simulink model "inverter_simulation"  (R2024b)
settings: Solver=VariableStepAuto  StartTime=0.0  StopTime=2  RelTol=1e-3
values from neighbouring files (symbols this model uses):
  Cdc = 2200e-6    (= 0.0022)    [parameters.m]
  KI_curr_d = KP_curr_d * Wp1_in    [pi_tuning.m]
  KI_curr_q = KI_curr_d    [pi_tuning.m]
  KI_q = C_q_ctrl.Ki    [pi_tuning.m]
  KI_volt = C_volt.Ki    [pi_tuning.m]
  KP_curr_d = Wbi / (DCGain_id * Wp1_in)    [pi_tuning.m]
  KP_curr_q = KP_curr_d    [pi_tuning.m]
  KP_q = C_q_ctrl.Kp    [pi_tuning.m]
  KP_volt = C_volt.Kp    [pi_tuning.m]
  Lc = 2.54e-3    (= 0.00254)    [parameters.m]
  P = 0.041    [parameters.m]
  rac = 1e-3    (= 0.001)    [parameters.m]
  rdc = Vdc^2 / P    (= 21951.2195122)    [parameters.m]
  Vdc = 30    [parameters.m]
  Vs = 20/sqrt(2)    [parameters.m]
  Zl = w * Lc    (= 0.957557440814)    [parameters.m]
libraries: slpidlib x4, spsMosfetLib x4, spsSeriesRLCBranchLib x3, spsVoltageMeasurementLib x3, spsCurrentMeasurementLib x2, spsACVoltageSourceLib x1, spsParallelRLCBranchLib x1, spsGroundLib x1, spsPWMGenerator2LevelLib x1, eePowerMeasurement x1, spspowerguiLib x1
settings Model: Creator=Asus  LastModifiedBy=Asus
settings RTWCC: GenCodeOnly=on

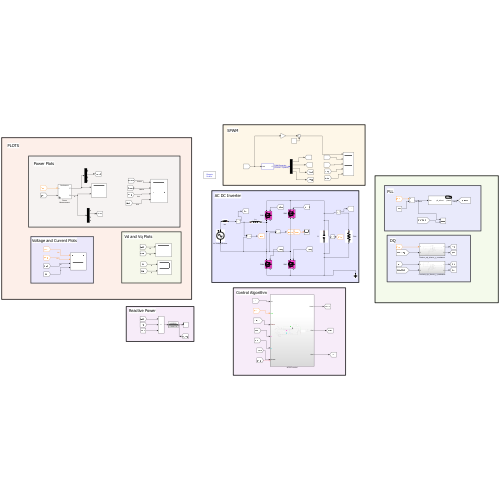
[thumbnail: Simulink's stored preview of the top-level diagram]
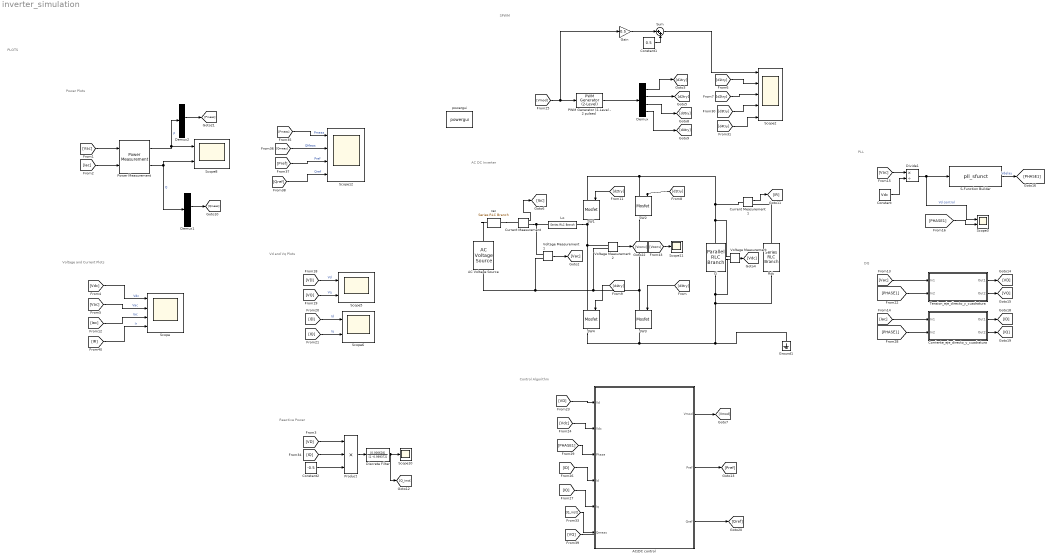
== system inverter_simulation ==
  note: PLL
  note: SPWM
  note: PLOTS
  note: Control Algorithm
  note: AC DC Inverter
  note: Power Plots
  note: Voltage and Current Plots
  note: Vd and Vq Plots
  note: DQ
  note: Reactive Power
  AC Voltage Source : spsACVoltageSourceLib/AC Voltage Source  Amplitude=Vs*sqrt(2)  Phase=0  Frequency=60  SampleTime=0  Measurements=None  BusType=swing  Pref=10e3  Qref=0  Qmin=-inf  Qmax=+inf
  AC/DC control : Subsystem
  Ci : spsParallelRLCBranchLib/Parallel RLC Branch  LConnTagsString=a  RConnTagsString=__new0  BranchType=C  Resistance=1  Inductance=1e-3  SetiL0=off  InitialCurrent=0  Capacitance=Cdc  Setx0=on  InitialVoltage=20  Measurements=None
  Constant : Constant  Value=Vdc
  Constant1 : Constant  Value=0.5
  Constant2 : Constant  Value=-0.5
  Corriente_eje_directo_y_cuadratura : Subsystem
  Current Measurement : spsCurrentMeasurementLib/Current Measurement  PhasorSimulation=off  OutputType=Complex  PSBequivalent=0
  Current Measurement1 : spsCurrentMeasurementLib/Current Measurement  PhasorSimulation=off  OutputType=Complex  PSBequivalent=0
  Demux : Demux
  Demux1 : Demux
  Demux2 : Demux
  Discrete Filter : DiscreteFilter  Numerator=[0.000628]  Denominator=[1 -0.999372]
  Divide1 : Product  Inputs=*/
  Gain : Gain  Gain=0.5
  Ground1 : spsGroundLib/Ground  LConnTagsString=a
  Lo : spsSeriesRLCBranchLib/Series RLC Branch  LConnTagsString=__new0  RConnTagsString=__new0  BranchType=L  Resistance=rac  Inductance=Lc  SetiL0=off  InitialCurrent=Io0  Capacitance=1e-6  Setx0=off  InitialVoltage=0  Measurements=None
  PWM Generator (2-Level - 2 pulses) : spsPWMGenerator2LevelLib/PWM Generator (2-Level)  ModulatorType=Single-phase full-bridge - Bipolar modulation (4 pulses)  ModulatorMode=Unsynchronized  Fc=20000  Pc=0  nF=27  MinMax="[ -1  1 ]"  SamplingTechnique=Natural  ModulatingSignals=off  m=0.6  Freq=60  Phase=30  Ts=5e-6  ShowCarrierOutport=off
  Power Measurement : eePowerMeasurement/Power Measurement  LabelModeActiveChoice=Continuous  F=60  K=[0 1 2 3]  Ts=0
  Product : Product  Inputs=3
  Rdc : spsSeriesRLCBranchLib/Series RLC Branch  LConnTagsString=__new0  RConnTagsString=__new0  BranchType=R  Resistance=rdc  Inductance=1e-3  SetiL0=off  InitialCurrent=0  Capacitance=1e-6  Setx0=off  InitialVoltage=0  Measurements=None
  S-Function Builder : S-Function  FunctionName=pll_sfunct  SFunctionModules=pll_sfunct_wrapper.c  SFunctionDeploymentMode=off  EnableBusSupport=off  mask(S-Function Builder){}
      mask help: Simulink:masks:SFunctionBuilder_MD
      mask init:
      | val = [[.9  0.75 0.75 1 1 .9 .9 1]',[1 1 0.75 0.75 .9 .9 1 .9]'];try , sys = get_param(gcb,'SfunBuilderFcnName');if isempty(sys), sys = get_param(gcb,'FunctionName'); end,catch, sys = get_param(gcb,'FunctionName'); end
      settings: CopyFcn=set_param(gcbh,'LinkStatus','none')  OpenFcn=sfunctionwizard(gcbh)
      mask Display:
      | plot(val(:,1),val(:,2))
      | disp(sys)
      | port_label('input',1,sprintf('%s', 'Vac'),'interpreter','tex')
      | port_label('output',1,sprintf('%s', 'phase'),'interpreter','tex')
  SW{1..4} (4 alike) : spsMosfetLib/Mosfet  Ron=1e-3  Lon=0  Rd=0.00001  Vfd=0  IC=0  Rs=1e5  Cs=inf  Measurements=on
  Scope : Scope  NumInputPorts=4
  Scope10 : Scope
  Scope11 : Scope
  Scope12 : Scope  NumInputPorts=4
  Scope2 : Scope  NumInputPorts=5
  Scope{3,5..6,8} (4 alike) : Scope  NumInputPorts=2
  Sum : Sum  Inputs=|++
  Tension_eje_directo_y_cuadratura : Subsystem
  Voltage Measurement : spsVoltageMeasurementLib/Voltage Measurement  PhasorSimulation=off  OutputType=Complex  PSBequivalent=0
  Voltage Measurement1 : spsVoltageMeasurementLib/Voltage Measurement  PhasorSimulation=off  OutputType=Complex  PSBequivalent=0
  Voltage Measurement2 : spsVoltageMeasurementLib/Voltage Measurement  PhasorSimulation=off  OutputType=Complex  PSBequivalent=0
  powergui : spspowerguiLib/powergui  Priority=1  SimulationMode=Discrete  SampleTime=5e-6  frequency=60  Iterations=50  frequencyindice=60  Pbase=100e6  ErrMax=1e-4  UnitsV=kV  UnitsW=MW  buscounter=0  FunctionMessages=off  echomessages=off  EnableUseOfTLC=off  CurrentSourceSwitches=off  DisableSnubberDevices=off  DisableRonSwitches=off  DisableVfSwitches=off  DisplayEquations=off  AutomaticDiscreteSolvers=off  SolverType=Tustin/Backward Euler (TBE)  Interpol=off  ExternalGateDelay=off  methode=off  Ts=100  x0status=blocks  SPID=on  SwTol=0  HookPort=off  NonlinearTolerance=1e-4  nMaxIteration=100  ContinueOnMaxIteration=off  RestoreLinks=warning  ResistiveCurrentMeasurement=off  Frange=[0:2:500]  Ylog=off  Xlog=on  ShowGrid=off  save=off  variable=ZData  structure=0  ZoomFFT=off  StartTime=0.0  cycles=1  DisplayStyle=1  fundamental=60  FreqAxis=off  MaxFrequency=1000  frequencyindicesteady=1  RmsSteady=1  display=off
  rac : spsSeriesRLCBranchLib/Series RLC Branch  LConnTagsString=__new0  RConnTagsString=__new0  BranchType=R  Resistance=rac  Inductance=Lc  SetiL0=off  InitialCurrent=Io0  Capacitance=1e-6  Setx0=off  InitialVoltage=0  Measurements=None
  wires:
  Voltage Measurement/1 -> [Vdc]
  PWM Generator (2-Level - 2 pulses)/1 -> Demux/1
  Demux/1 -> [d1try]
  Demux/2 -> [d2try]
  [d1try] -> Scope2/2
  [d2try] -> Scope2/3
  Current Measurement/1 -> [Iac]
  Tension_eje_directo_y_cuadratura/1(Out1) -> [VD]
  Corriente_eje_directo_y_cuadratura/1(Out1) -> [ID]
  Tension_eje_directo_y_cuadratura/2(Out2) -> [VQ]
  [Iac] -> Corriente_eje_directo_y_cuadratura/1(In1)
  [Vac] -> Tension_eje_directo_y_cuadratura/1(In1)
  [PHASE1] -> Corriente_eje_directo_y_cuadratura/2(In2)
  Corriente_eje_directo_y_cuadratura/2(Out2) -> [IQ]
  [PHASE1] -> Tension_eje_directo_y_cuadratura/2(In2)
  [PHASE1] -> Scope3/2
  [VD] -> Scope5/1  "Vd"
  [VQ] -> Scope5/2  "Vq"
  [ID] -> Scope6/1  "Id"
  [IQ] -> Scope6/2  "Iq"
  [VD] -> AC/DC control/1(Vd)
  [Vdc] -> AC/DC control/2(Vdc)
  AC/DC control/1(Vmod) -> [Vmod]
  [PHASE1] -> AC/DC control/3(Phase)
  [Vac] -> Divide1/1
  Divide1/1 -> Scope3/1, S-Function Builder/1  "Vd control"
  Constant/1 -> Divide1/2
  Demux/3 -> [d3try]
  Demux/4 -> [d4try]
  [d3try] -> Scope2/4
  [d4try] -> Scope2/5
  Voltage Measurement1/1 -> [Vac]
  [ID] -> AC/DC control/4(Id)
  [IQ] -> AC/DC control/5(Iq)
  Current Measurement1/1 -> [IR]
  Voltage Measurement2/1 -> [Vconv]
  [Vconv] -> Scope11/1
  [d1try] -> SW2/1
  [d2try] -> SW1/1
  [d4try] -> SW4/1
  Gain/1 -> Sum/1
  Constant1/1 -> Sum/2
  Sum/1 -> Scope2/1
  [d3try] -> SW3/1
  S-Function Builder/1 -> [PHASE1]  "Vdelay"
  Constant2/1 -> Product/3
  [IQ] -> Product/2
  Discrete Filter/1 -> [Q_inst], Scope10/1
  [VD] -> Product/1
  Product/1 -> Discrete Filter/1
  [Q_inst] -> AC/DC control/6(Qmeas)
  AC/DC control/2(Pref) -> [Pref]
  AC/DC control/3(Qref) -> [Qref]
  [VQ] -> ?
  [Vmod] -> Gain/1, PWM Generator (2-Level - 2 pulses)/1
  [IR] -> Scope/4  "Ir"
  [Pref] -> Scope12/3  "Pref"
  [Iac] -> Scope/3  "Iac"
  [Qref] -> Scope12/4  "Qref"
  [Qmeas] -> Scope12/2  "QMeas"
  [Vac] -> Scope/2  "Vac"
  [Vac] -> Power Measurement/1
  Power Measurement/1 -> Demux2/1, Scope8/1  "P"
  [Vdc] -> Scope/1  "Vdc"
  Power Measurement/2 -> Demux1/1, Scope8/2  "Q"
  [Iac] -> Power Measurement/2
  Demux1/2 -> [Qmeas]
  [Pmeas] -> Scope12/1  "Pmeas"
  Demux2/2 -> [Pmeas]
  connections:
  Current Measurement/RConn1 -- Voltage Measurement1/LConn1 -- Lo/LConn1
  SW1/LConn1 -- Ci/LConn1 -- Voltage Measurement/LConn1 -- Current Measurement1/LConn1 -- SW2/LConn1
  Ci/RConn1 -- Voltage Measurement/LConn2 -- SW3/RConn1 -- SW4/RConn1 -- Ground1/LConn1 -- Rdc/RConn1
  SW2/RConn1 -- Voltage Measurement2/LConn2 -- AC Voltage Source/LConn1 -- Voltage Measurement1/LConn2 -- SW3/LConn1
  Lo/RConn1 -- Voltage Measurement2/LConn1 -- SW4/LConn1 -- SW1/RConn1
  rac/RConn1 -- AC Voltage Source/RConn1
  rac/LConn1 -- Current Measurement/LConn1
  Rdc/LConn1 -- Current Measurement1/RConn1

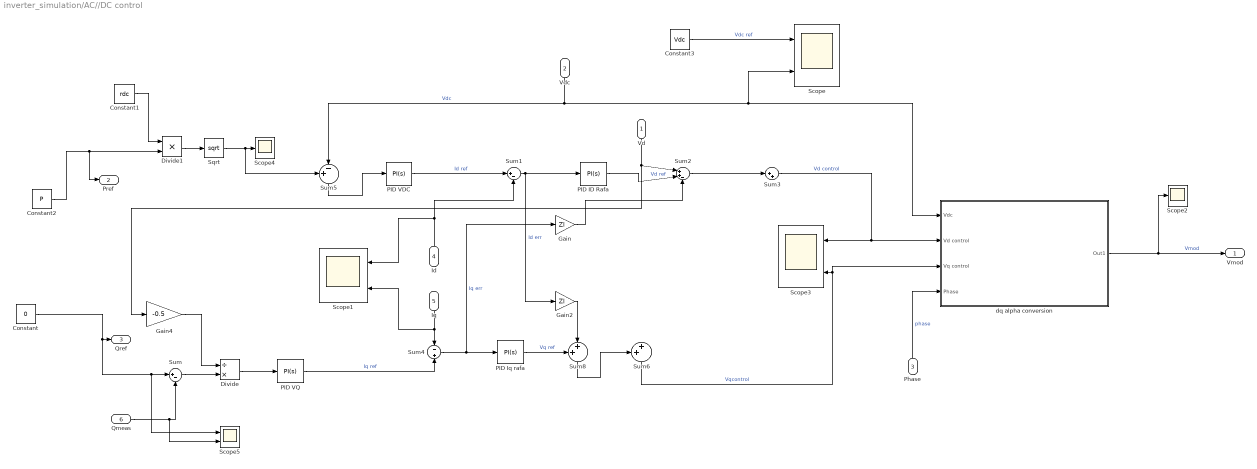
== system inverter_simulation/AC//DC control ==
  Vd : Inport
  Vdc : Inport  Port=2
  Phase : Inport  Port=3
  Id : Inport  Port=4
  Iq : Inport  Port=5
  Qmeas : Inport  Port=6
  Constant : Constant  Value=0
  Constant1 : Constant  Value=rdc
  Constant2 : Constant  Value=P
  Constant3 : Constant  Value=Vdc
  Divide : Product  Inputs=/*
  Divide1 : Product  Inputs=**
  Gain : Gain  Gain=Zl
  Gain2 : Gain  Gain=Zl
  Gain4 : Gain  Gain=-0.5
  PID ID Rafa : slpidlib/PID Controller  Controller=PI  Form=Parallel  TimeDomain=Continuous-time  UseExternalTs=off  SampleTime=-1  IntegratorMethod=Forward Euler  FilterMethod=Forward Euler  ControllerParametersSource=internal  P=KP_curr_d  I=KI_curr_d  UseKiTs=off  D=0  UseExternalDerivativeSource=off  N=100  UseFilter=on  TunerSelectOption=Transfer Function Based (PID Tuner App)  InitialConditionSource=internal  InitialConditionForIntegrator=0  InitialConditionForFilter=0  DifferentiatorICPrevScaledInput=0  ExternalReset=none  TrackingMode=off  Kt=1  LimitOutput=off  SatLimitsSource=internal  UpperSaturationLimit=200  LowerSaturationLimit=-inf  LinearizeAsGain=on  AntiWindupMode=none  Kb=1  LimitIntegrator=off  UpperIntegratorSaturationLimit=inf  LowerIntegratorSaturationLimit=-inf  POutMin=[]  POutMax=[]  IOutMin=[]  IOutMax=[]  DOutMin=[]  DOutMax=[]  NOutMin=[]  NOutMax=[]  SumOutMin=[]  SumOutMax=[]  SaturationOutMin=[]  SaturationOutMax=[]  PParamMin=[]  PParamMax=[]  IParamMin=[]  IParamMax=[]  DParamMin=[]  DParamMax=[]  NParamMin=[]  NParamMax=[]  KbParamMin=[]  KbParamMax=[]  KtParamMin=[]  KtParamMax=[]  KbOutMin=[]  KbOutMax=[]  KtOutMin=[]  KtOutMax=[]  IntegratorOutMin=[]  IntegratorOutMax=[]  FilterOutMin=[]  FilterOutMax=[]  SumI1OutMin=[]  SumI1OutMax=[]  SumI2OutMin=[]  SumI2OutMax=[]  SumI3OutMin=[]  SumI3OutMax=[]  SumI4OutMin=[]  SumI4OutMax=[]  SumDOutMin=[]  SumDOutMax=[]  DifferentiatorOutMin=[]  DifferentiatorOutMax=[]  FilterDiffOutCoefMin=[]  FilterDiffOutCoefMax=[]  ReciprocalOutMin=[]  ReciprocalOutMax=[]  SumDenOutMin=[]  SumDenOutMax=[]  SumNumOutMin=[]  SumNumOutMax=[]  DivideOutMin=[]  DivideOutMax=[]  UdiffTsProdOutMin=[]  UdiffTsProdOutMax=[]  NTsProdOutMin=[]  NTsProdOutMax=[]  UintegralTsProdOutMin=[]  UintegralTsProdOutMax=[]  UngainTsProdOutMin=[]  UngainTsProdOutMax=[]  ClampingZeroOutDataTypeStr=Inherit: Inherit via back propagation  ClampingZeroOutMin=[]  ClampingZeroOutMax=[]  FilterDenConstantOutDataTypeStr=Inherit: Inherit via back propagation  FilterDenConstantOutMin=[]  FilterDenConstantOutMax=[]  PCopyOutDataTypeStr=Inherit: Inherit via back propagation  PCopyOutMin=[]  PCopyOutMax=[]  NCopyOutDataTypeStr=Inherit: Inherit via back propagation  NCopyOutMin=[]  NCopyOutMax=[]  IntegratorContinuousStateAttributes=''  IntegratorStateMustResolveToSignalObject=off  IntegratorRTWStateStorageClass=Auto  FilterContinuousStateAttributes=''  FilterStateMustResolveToSignalObject=off  FilterRTWStateStorageClass=Auto  ParallelPVariant=InternalParameters  IdealPVariant=Disabled  IVariant=InternalParameters  DVariant=Disabled  IntegratorVariant=Continuous  SatVariant=Disabled  AWVariant=Passthrough  PCopyVariant=Disabled  TRVariant=Disabled  FdbkBlocksVariant=Forward  IdealPFdbkVariant=Disabled  SatFdbkVariant=Disabled  DerivativeFilterVariant=Disabled  NVariant=Disabled  NCopyVariant=Disabled_SignalSpec  FilterICVariant=Disabled  IntegratorICVariant=InternalICs  ExternalResetVariant=Disabled  TRSumVariant=Passthrough  SumFdbkVariant=Disabled  SumVariant=Sum_PI  TsampFilterVariant=InternalTs  TsampNgainVariant=Passthrough  TsampIntegralVariant=Disabled_SignalSpec  ExternalSaturationOutDataTypeStr=Inherit: Same as second input  DerivativeSourceVariant=Disabled  PreIntVariant=InternalPreInt
  PID Iq rafa : slpidlib/PID Controller  Controller=PI  Form=Parallel  TimeDomain=Continuous-time  UseExternalTs=off  SampleTime=-1  IntegratorMethod=Forward Euler  FilterMethod=Forward Euler  ControllerParametersSource=internal  P=KP_curr_q  I=KI_curr_q  UseKiTs=off  D=0  UseExternalDerivativeSource=off  N=100  UseFilter=on  TunerSelectOption=Transfer Function Based (PID Tuner App)  InitialConditionSource=internal  InitialConditionForIntegrator=0  InitialConditionForFilter=0  DifferentiatorICPrevScaledInput=0  ExternalReset=none  TrackingMode=off  Kt=1  LimitOutput=off  SatLimitsSource=internal  UpperSaturationLimit=15  LowerSaturationLimit=-15  LinearizeAsGain=on  AntiWindupMode=none  Kb=1  LimitIntegrator=off  UpperIntegratorSaturationLimit=inf  LowerIntegratorSaturationLimit=-inf  POutMin=[]  POutMax=[]  IOutMin=[]  IOutMax=[]  DOutMin=[]  DOutMax=[]  NOutMin=[]  NOutMax=[]  SumOutMin=[]  SumOutMax=[]  SaturationOutMin=[]  SaturationOutMax=[]  PParamMin=[]  PParamMax=[]  IParamMin=[]  IParamMax=[]  DParamMin=[]  DParamMax=[]  NParamMin=[]  NParamMax=[]  KbParamMin=[]  KbParamMax=[]  KtParamMin=[]  KtParamMax=[]  KbOutMin=[]  KbOutMax=[]  KtOutMin=[]  KtOutMax=[]  IntegratorOutMin=[]  IntegratorOutMax=[]  FilterOutMin=[]  FilterOutMax=[]  SumI1OutMin=[]  SumI1OutMax=[]  SumI2OutMin=[]  SumI2OutMax=[]  SumI3OutMin=[]  SumI3OutMax=[]  SumI4OutMin=[]  SumI4OutMax=[]  SumDOutMin=[]  SumDOutMax=[]  DifferentiatorOutMin=[]  DifferentiatorOutMax=[]  FilterDiffOutCoefMin=[]  FilterDiffOutCoefMax=[]  ReciprocalOutMin=[]  ReciprocalOutMax=[]  SumDenOutMin=[]  SumDenOutMax=[]  SumNumOutMin=[]  SumNumOutMax=[]  DivideOutMin=[]  DivideOutMax=[]  UdiffTsProdOutMin=[]  UdiffTsProdOutMax=[]  NTsProdOutMin=[]  NTsProdOutMax=[]  UintegralTsProdOutMin=[]  UintegralTsProdOutMax=[]  UngainTsProdOutMin=[]  UngainTsProdOutMax=[]  ClampingZeroOutDataTypeStr=Inherit: Inherit via back propagation  ClampingZeroOutMin=[]  ClampingZeroOutMax=[]  FilterDenConstantOutDataTypeStr=Inherit: Inherit via back propagation  FilterDenConstantOutMin=[]  FilterDenConstantOutMax=[]  PCopyOutDataTypeStr=Inherit: Inherit via back propagation  PCopyOutMin=[]  PCopyOutMax=[]  NCopyOutDataTypeStr=Inherit: Inherit via back propagation  NCopyOutMin=[]  NCopyOutMax=[]  IntegratorContinuousStateAttributes=''  IntegratorStateMustResolveToSignalObject=off  IntegratorRTWStateStorageClass=Auto  FilterContinuousStateAttributes=''  FilterStateMustResolveToSignalObject=off  FilterRTWStateStorageClass=Auto  ParallelPVariant=InternalParameters  IdealPVariant=Disabled  IVariant=InternalParameters  DVariant=Disabled  IntegratorVariant=Continuous  SatVariant=Disabled  AWVariant=Passthrough  PCopyVariant=Disabled  TRVariant=Disabled  FdbkBlocksVariant=Forward  IdealPFdbkVariant=Disabled  SatFdbkVariant=Disabled  DerivativeFilterVariant=Disabled  NVariant=Disabled  NCopyVariant=Disabled_SignalSpec  FilterICVariant=Disabled  IntegratorICVariant=InternalICs  ExternalResetVariant=Disabled  TRSumVariant=Passthrough  SumFdbkVariant=Disabled  SumVariant=Sum_PI  TsampFilterVariant=InternalTs  TsampNgainVariant=Passthrough  TsampIntegralVariant=Disabled_SignalSpec  ExternalSaturationOutDataTypeStr=Inherit: Same as second input  DerivativeSourceVariant=Disabled  PreIntVariant=InternalPreInt
  PID VDC : slpidlib/PID Controller  Controller=PI  Form=Parallel  TimeDomain=Continuous-time  UseExternalTs=off  SampleTime=-1  IntegratorMethod=Forward Euler  FilterMethod=Forward Euler  ControllerParametersSource=internal  P=-KP_volt  I=-KI_volt  UseKiTs=off  D=0  UseExternalDerivativeSource=off  N=100  UseFilter=on  TunerSelectOption=Frequency Response Based  InitialConditionSource=internal  InitialConditionForIntegrator=0  InitialConditionForFilter=0  DifferentiatorICPrevScaledInput=0  ExternalReset=none  TrackingMode=off  Kt=1  LimitOutput=off  SatLimitsSource=internal  UpperSaturationLimit=16  LowerSaturationLimit=-16  LinearizeAsGain=on  AntiWindupMode=none  Kb=1  LimitIntegrator=off  UpperIntegratorSaturationLimit=inf  LowerIntegratorSaturationLimit=-inf  POutMin=[]  POutMax=[]  IOutMin=[]  IOutMax=[]  DOutMin=[]  DOutMax=[]  NOutMin=[]  NOutMax=[]  SumOutMin=[]  SumOutMax=[]  SaturationOutMin=[]  SaturationOutMax=[]  PParamMin=[]  PParamMax=[]  IParamMin=[]  IParamMax=[]  DParamMin=[]  DParamMax=[]  NParamMin=[]  NParamMax=[]  KbParamMin=[]  KbParamMax=[]  KtParamMin=[]  KtParamMax=[]  KbOutMin=[]  KbOutMax=[]  KtOutMin=[]  KtOutMax=[]  IntegratorOutMin=[]  IntegratorOutMax=[]  FilterOutMin=[]  FilterOutMax=[]  SumI1OutMin=[]  SumI1OutMax=[]  SumI2OutMin=[]  SumI2OutMax=[]  SumI3OutMin=[]  SumI3OutMax=[]  SumI4OutMin=[]  SumI4OutMax=[]  SumDOutMin=[]  SumDOutMax=[]  DifferentiatorOutMin=[]  DifferentiatorOutMax=[]  FilterDiffOutCoefMin=[]  FilterDiffOutCoefMax=[]  ReciprocalOutMin=[]  ReciprocalOutMax=[]  SumDenOutMin=[]  SumDenOutMax=[]  SumNumOutMin=[]  SumNumOutMax=[]  DivideOutMin=[]  DivideOutMax=[]  UdiffTsProdOutMin=[]  UdiffTsProdOutMax=[]  NTsProdOutMin=[]  NTsProdOutMax=[]  UintegralTsProdOutMin=[]  UintegralTsProdOutMax=[]  UngainTsProdOutMin=[]  UngainTsProdOutMax=[]  ClampingZeroOutDataTypeStr=Inherit: Inherit via back propagation  ClampingZeroOutMin=[]  ClampingZeroOutMax=[]  FilterDenConstantOutDataTypeStr=Inherit: Inherit via back propagation  FilterDenConstantOutMin=[]  FilterDenConstantOutMax=[]  PCopyOutDataTypeStr=Inherit: Inherit via back propagation  PCopyOutMin=[]  PCopyOutMax=[]  NCopyOutDataTypeStr=Inherit: Inherit via back propagation  NCopyOutMin=[]  NCopyOutMax=[]  IntegratorContinuousStateAttributes=''  IntegratorStateMustResolveToSignalObject=off  IntegratorRTWStateStorageClass=Auto  FilterContinuousStateAttributes=''  FilterStateMustResolveToSignalObject=off  FilterRTWStateStorageClass=Auto  ParallelPVariant=InternalParameters  IdealPVariant=Disabled  IVariant=InternalParameters  DVariant=Disabled  IntegratorVariant=Continuous  SatVariant=Disabled  AWVariant=Passthrough  PCopyVariant=Disabled  TRVariant=Disabled  FdbkBlocksVariant=Forward  IdealPFdbkVariant=Disabled  SatFdbkVariant=Disabled  DerivativeFilterVariant=Disabled  NVariant=Disabled  NCopyVariant=Disabled_SignalSpec  FilterICVariant=Disabled  IntegratorICVariant=InternalICs  ExternalResetVariant=Disabled  TRSumVariant=Passthrough  SumFdbkVariant=Disabled  SumVariant=Sum_PI  TsampFilterVariant=InternalTs  TsampNgainVariant=Passthrough  TsampIntegralVariant=Disabled_SignalSpec  ExternalSaturationOutDataTypeStr=Inherit: Same as second input  DerivativeSourceVariant=Disabled  PreIntVariant=InternalPreInt
  PID VQ : slpidlib/PID Controller  Controller=PI  Form=Parallel  TimeDomain=Continuous-time  UseExternalTs=off  SampleTime=-1  IntegratorMethod=Forward Euler  FilterMethod=Forward Euler  ControllerParametersSource=internal  P=KP_q+0.08  I=KI_q  UseKiTs=off  D=0  UseExternalDerivativeSource=off  N=100  UseFilter=on  TunerSelectOption=Frequency Response Based  InitialConditionSource=internal  InitialConditionForIntegrator=0  InitialConditionForFilter=0  DifferentiatorICPrevScaledInput=0  ExternalReset=none  TrackingMode=off  Kt=1  LimitOutput=off  SatLimitsSource=internal  UpperSaturationLimit=16  LowerSaturationLimit=-16  LinearizeAsGain=on  AntiWindupMode=none  Kb=1  LimitIntegrator=off  UpperIntegratorSaturationLimit=inf  LowerIntegratorSaturationLimit=-inf  POutMin=[]  POutMax=[]  IOutMin=[]  IOutMax=[]  DOutMin=[]  DOutMax=[]  NOutMin=[]  NOutMax=[]  SumOutMin=[]  SumOutMax=[]  SaturationOutMin=[]  SaturationOutMax=[]  PParamMin=[]  PParamMax=[]  IParamMin=[]  IParamMax=[]  DParamMin=[]  DParamMax=[]  NParamMin=[]  NParamMax=[]  KbParamMin=[]  KbParamMax=[]  KtParamMin=[]  KtParamMax=[]  KbOutMin=[]  KbOutMax=[]  KtOutMin=[]  KtOutMax=[]  IntegratorOutMin=[]  IntegratorOutMax=[]  FilterOutMin=[]  FilterOutMax=[]  SumI1OutMin=[]  SumI1OutMax=[]  SumI2OutMin=[]  SumI2OutMax=[]  SumI3OutMin=[]  SumI3OutMax=[]  SumI4OutMin=[]  SumI4OutMax=[]  SumDOutMin=[]  SumDOutMax=[]  DifferentiatorOutMin=[]  DifferentiatorOutMax=[]  FilterDiffOutCoefMin=[]  FilterDiffOutCoefMax=[]  ReciprocalOutMin=[]  ReciprocalOutMax=[]  SumDenOutMin=[]  SumDenOutMax=[]  SumNumOutMin=[]  SumNumOutMax=[]  DivideOutMin=[]  DivideOutMax=[]  UdiffTsProdOutMin=[]  UdiffTsProdOutMax=[]  NTsProdOutMin=[]  NTsProdOutMax=[]  UintegralTsProdOutMin=[]  UintegralTsProdOutMax=[]  UngainTsProdOutMin=[]  UngainTsProdOutMax=[]  ClampingZeroOutDataTypeStr=Inherit: Inherit via back propagation  ClampingZeroOutMin=[]  ClampingZeroOutMax=[]  FilterDenConstantOutDataTypeStr=Inherit: Inherit via back propagation  FilterDenConstantOutMin=[]  FilterDenConstantOutMax=[]  PCopyOutDataTypeStr=Inherit: Inherit via back propagation  PCopyOutMin=[]  PCopyOutMax=[]  NCopyOutDataTypeStr=Inherit: Inherit via back propagation  NCopyOutMin=[]  NCopyOutMax=[]  IntegratorContinuousStateAttributes=''  IntegratorStateMustResolveToSignalObject=off  IntegratorRTWStateStorageClass=Auto  FilterContinuousStateAttributes=''  FilterStateMustResolveToSignalObject=off  FilterRTWStateStorageClass=Auto  ParallelPVariant=InternalParameters  IdealPVariant=Disabled  IVariant=InternalParameters  DVariant=Disabled  IntegratorVariant=Continuous  SatVariant=Disabled  AWVariant=Passthrough  PCopyVariant=Disabled  TRVariant=Disabled  FdbkBlocksVariant=Forward  IdealPFdbkVariant=Disabled  SatFdbkVariant=Disabled  DerivativeFilterVariant=Disabled  NVariant=Disabled  NCopyVariant=Disabled_SignalSpec  FilterICVariant=Disabled  IntegratorICVariant=InternalICs  ExternalResetVariant=Disabled  TRSumVariant=Passthrough  SumFdbkVariant=Disabled  SumVariant=Sum_PI  TsampFilterVariant=InternalTs  TsampNgainVariant=Passthrough  TsampIntegralVariant=Disabled_SignalSpec  ExternalSaturationOutDataTypeStr=Inherit: Same as second input  DerivativeSourceVariant=Disabled  PreIntVariant=InternalPreInt
  Scope{,1,3,5} (4 alike) : Scope  NumInputPorts=2
  Scope2 : Scope
  Scope4 : Scope
  Sqrt : Sqrt
  Sum : Sum  Inputs=|+-
  Sum1 : Sum  Inputs=|+-
  Sum2 : Sum  Inputs=|++-
  Sum3 : Sum  Inputs=|++
  Sum4 : Sum  Inputs=-+
  Sum5 : Sum  Inputs=+-|
  Sum6 : Sum  Inputs=++|
  Sum8 : Sum  Inputs=++|
  dq alpha conversion : Subsystem
  Vmod : Outport
  Pref : Outport  Port=2
  Qref : Outport  Port=3
  wires:
  Sum4/1 -> PID Iq rafa/1, Gain/1  "Iq err"
  Sum8/1 -> Sum6/1
  Sum1/1 -> PID ID Rafa/1, Gain2/1  "Id err"
  Sum2/1 -> Sum3/1
  PID Iq rafa/1 -> Sum8/1  "Vq ref"
  Phase/1 -> dq alpha conversion/4(Phase)  "phase"
  PID ID Rafa/1 -> Sum2/2  "Vd ref"
  Vdc/1 -> Scope/2, dq alpha conversion/1(Vdc), Sum5/2  "Vdc"
  dq alpha conversion/1(Out1) -> Scope2/1, Vmod/1  "Vmod"
  Sum5/1 -> PID VDC/1
  Gain/1 -> Sum2/3
  Gain2/1 -> Sum8/2
  Id/1 -> Scope1/1, Sum1/2
  Iq/1 -> Scope1/2, Sum4/1
  Sum3/1 -> Scope3/1, dq alpha conversion/2(Vd control)  "Vd control"
  Sum6/1 -> dq alpha conversion/3(Vq control), Scope3/2  "Vqcontrol"
  Constant3/1 -> Scope/1  "Vdc ref"
  Vd/1 -> Gain4/1, Sum2/1
  Divide/1 -> PID VQ/1
  Qmeas/1 -> Scope5/2, Sum/2
  Sum/1 -> Divide/2
  Gain4/1 -> Divide/1
  Constant/1 -> Scope5/1, Sum/1, Qref/1
  Constant2/1 -> Pref/1, Divide1/2
  Constant1/1 -> Divide1/1
  Divide1/1 -> Sqrt/1
  Sqrt/1 -> Sum5/1, Scope4/1
  PID VQ/1 -> Sum4/2  "Iq ref"
  PID VDC/1 -> Sum1/1  "Id ref"

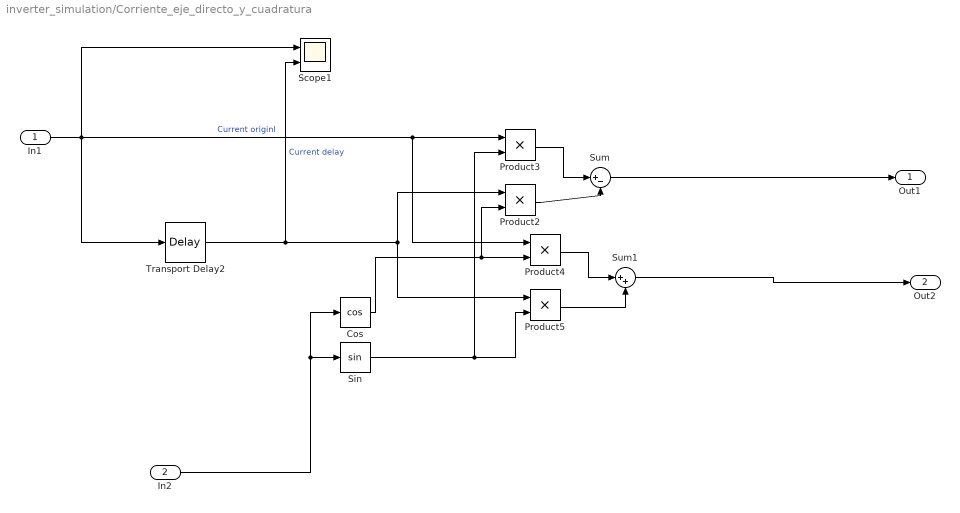
== system inverter_simulation/Corriente_eje_directo_y_cuadratura ==
  In1 : Inport
  In2 : Inport  Port=2
  Cos : Trigonometry  Operator=cos
  Product{2..5} (4 alike) : Product
  Scope1 : Scope  NumInputPorts=2
  Sin : Trigonometry
  Sum : Sum  Inputs=|+-
  Sum1 : Sum  Inputs=|++
  Transport Delay2 : TransportDelay  DelayTime=0.25/60
  Out1 : Outport
  Out2 : Outport  Port=2
  wires:
  In2/1 -> Sin/1, Cos/1
  Product4/1 -> Sum1/1
  Product3/1 -> Sum/1
  Product5/1 -> Sum1/2
  Sin/1 -> Product5/2, Product3/2
  Sum/1 -> Out1/1
  Sum1/1 -> Out2/1
  In1/1 -> Transport Delay2/1, Product3/1, Product4/1, Scope1/1  "Current originl"
  Transport Delay2/1 -> Scope1/2, Product5/1, Product2/1  "Current delay"
  Cos/1 -> Product2/2, Product4/2
  Product2/1 -> Sum/2

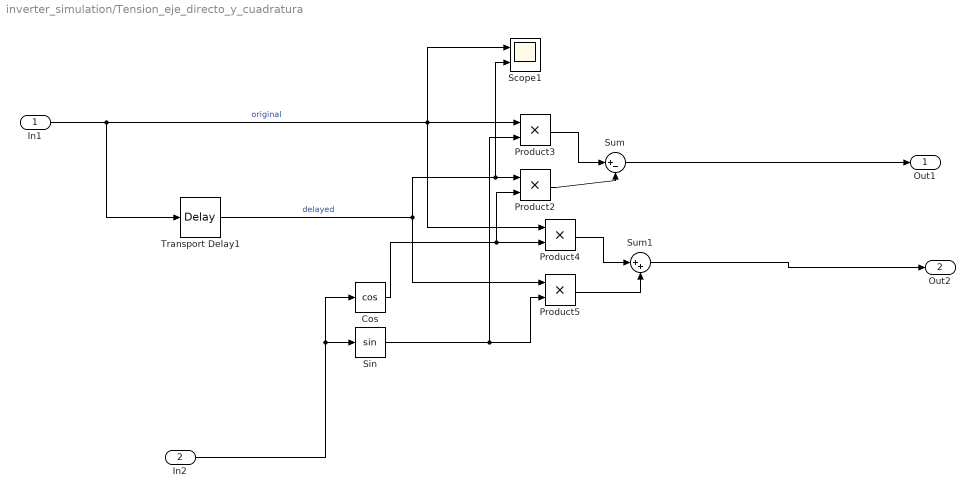
== system inverter_simulation/Tension_eje_directo_y_cuadratura ==
  In1 : Inport
  In2 : Inport  Port=2
  Cos : Trigonometry  Operator=cos
  Product{2..5} (4 alike) : Product
  Scope1 : Scope  NumInputPorts=2
  Sin : Trigonometry
  Sum : Sum  Inputs=|+-
  Sum1 : Sum  Inputs=|++
  Transport Delay1 : TransportDelay  DelayTime=0.25/60
  Out1 : Outport
  Out2 : Outport  Port=2
  wires:
  Product2/1 -> Sum/2
  Cos/1 -> Product4/2, Product2/2
  Transport Delay1/1 -> Scope1/2, Product2/1, Product5/1  "delayed"
  In1/1 -> Transport Delay1/1, Product4/1, Product3/1, Scope1/1  "original"
  Sum1/1 -> Out2/1
  Sum/1 -> Out1/1
  Sin/1 -> Product3/2, Product5/2
  Product5/1 -> Sum1/2
  Product3/1 -> Sum/1
  Product4/1 -> Sum1/1
  In2/1 -> Cos/1, Sin/1

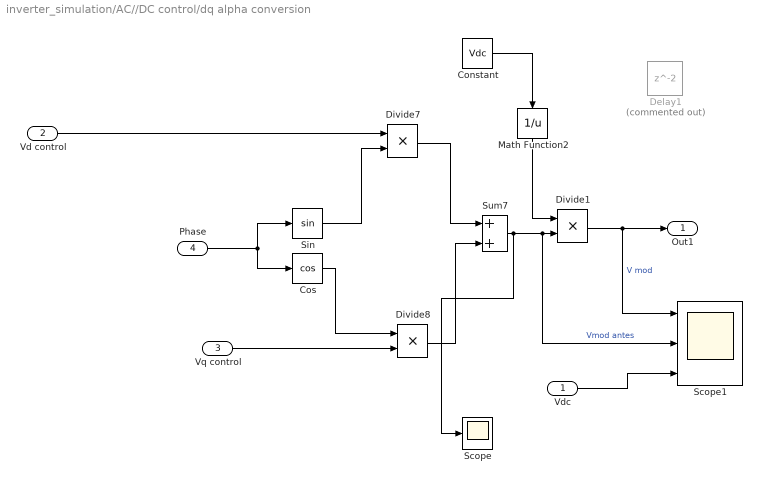
== system inverter_simulation/AC//DC control/dq alpha conversion ==
  Vdc : Inport
  Vd control : Inport  Port=2
  Vq control : Inport  Port=3
  Phase : Inport  Port=4
  Constant : Constant  Value=Vdc
  Cos : Trigonometry  Operator=cos
  Delay1 : Delay  Commented=on
  Divide1 : Product  Inputs=**
  Divide7 : Product  Inputs=**
  Divide8 : Product  Inputs=**
  Math Function2 : Math  Operator=reciprocal
  Scope : Scope
  Scope1 : Scope  NumInputPorts=3
  Sin : Trigonometry
  Sum7 : Sum
  Out1 : Outport
  wires:
  Cos/1 -> Divide8/1
  Sin/1 -> Divide7/2
  Vd control/1 -> Divide7/1
  Divide8/1 -> Sum7/2
  Divide7/1 -> Sum7/1
  Phase/1 -> Cos/1, Sin/1
  Vq control/1 -> Divide8/2
  Sum7/1 -> Scope/1, Scope1/2, Divide1/2  "Vmod antes"
  Divide1/1 -> Scope1/1, Out1/1  "V mod"
  Vdc/1 -> Scope1/3
  Math Function2/1 -> Divide1/1
  Constant/1 -> Math Function2/1
